simulink model "GATE_A"  (R2016a)
settings: Solver=FixedStepDiscrete  StartTime=0.0  StopTime=120  RelTol=1e-3
values from neighbouring files (symbols this model uses):
  CLOSE_CHAR = CHAR_STAR    [GateParameter.m]
  CLOSE_SIDE_VALUE = single(4*ONE_SEC)    [GateParameter.m]
  CLOSED = uint8(12)    [GateParameter.m]
  CLOSING = uint8(13)    [GateParameter.m]
  INIT = uint8(15)    [GateParameter.m]
  NO_PASS_ASSIG = uint8(6)    [GateParameter.m]
  OPEN = uint8(14)    [GateParameter.m]
  OPEN_CHAR = CHAR_HASH    [GateParameter.m]
  OPEN_SIDE_VALUE = uint16(4*ONE_SEC)    [GateParameter.m]
  OPENING = uint8(11)    [GateParameter.m]
  OPENING_ACTIVE = uint8(1)    [GateParameter.m]
  PASS_ASSIGNED = uint8(7)    [GateParameter.m]
  PASS_INCOMPLETE = uint8(8)    [GateParameter.m]
  PASS_TIMEOUT = uint16(10*ONE_SEC)    [GateParameter.m]
  PASSWORD_VERIFIED = uint8(5)    [GateParameter.m]
  TIMEOUT = uint8(9)    [GateParameter.m]
  WRONG_PASSWORD = uint8(2)    [GateParameter.m]
undefined symbols (not defined in the file or in its folder): OPEN_TIMEOUT
(part 2 of 2)

== stateflow chart GATE_A/A_HardwareOutputWrapper_BT_KP_RF/BT_TxHandler/BT_TxHandler ==
  state Idle
    entry:
    BT_TxChar_UINT8 = 0;
  state WrongPass
    entry:
    BT_TxChar_UINT8 = 119;
    counter = 0;
    du:
    counter++;
  state BtInput
  state sendClose
    entry:
    BT_TxChar_UINT8 = 99;
  state sendOpen
    entry:
    BT_TxChar_UINT8 = 98;
  state sendOpening
    entry:
    BT_TxChar_UINT8 = 97;
  (default) -> Idle
  Idle -> (junction 8) : [hasChanged(BTCharReceived)]
  (junction 8) -> BtInput : [BTCharReceived != 0]
  sendClose -> Idle : [leftMotor == CLOSED]
  WrongPass -> Idle : [counter >= 10]
  BtInput -> WrongPass [order 2] : [PassSuccess == WRONG_PASSWORD]
  BtInput -> sendOpening [order 1] : [leftMotor == OPENING]
  sendOpen -> sendClose : [rightMotor == CLOSING]
  sendOpening -> sendOpen : [rightMotor == OPEN]
  data: BTCharReceived input; leftMotor input; rightMotor input; BT_TxChar_UINT8 output uint8; PassSuccess input; CLOSED input; CLOSING input; OPEN input; OPENING input; WRONG_PASSWORD input; counter local uint8
